simulink model "untitled"  (R2025b)
settings: Solver=VariableStepAuto  StartTime=0.0  StopTime=0.5  FixedStep=1e-5  RelTol=1e-3
libraries: fl_lib x17, nesl_utility x7, eeGeneralControl x2, eePowerMeasurement x1
settings Model: Creator=lenovo  LastModifiedBy=lenovo

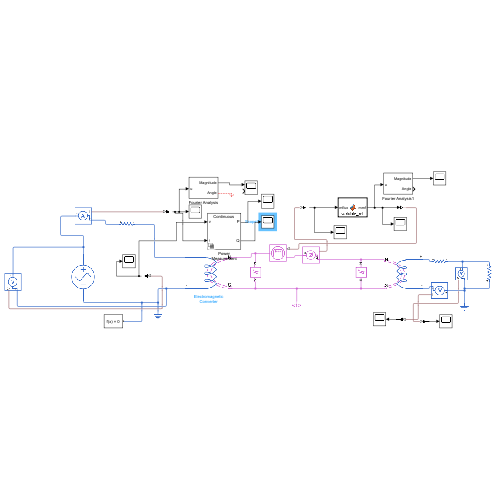
[thumbnail: Simulink's stored preview of the top-level diagram]
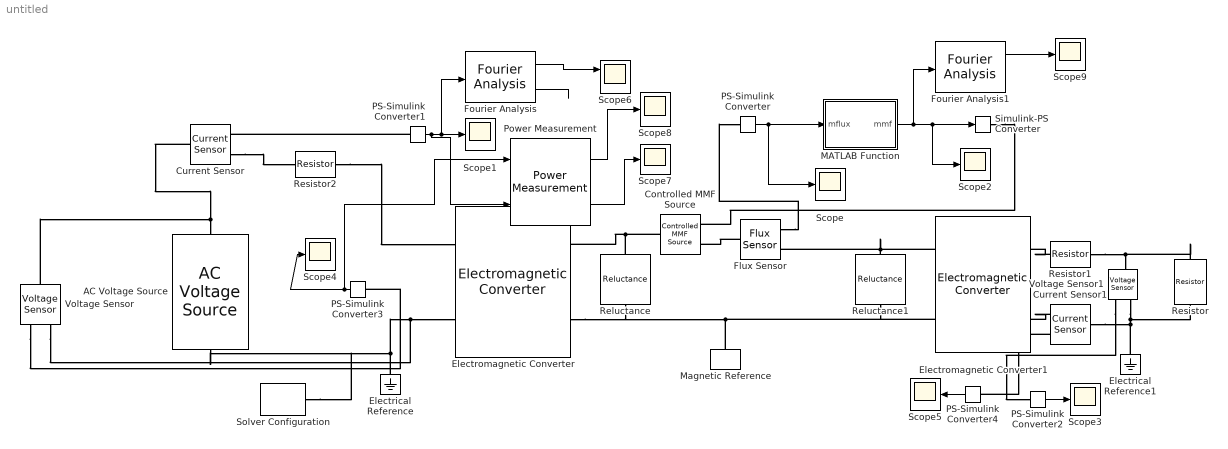
== system untitled ==
  AC Voltage Source : fl_lib/Electrical/Electrical Sources/AC Voltage Source  amp=49.9 V  shift=90 deg  frequency=50 Hz
  Controlled MMF Source : fl_lib/Magnetic/Magnetic Sources/Controlled MMF Source
      settings: InternalSimscapePortConfiguration="{\"Bottom\":[],\"Left\":[{\"id\":\"N\",\"label\":\"\",\"type\":\"foundation.magnetic.magnetic\"}],\"Right\":[{\"id\":\"mmfI\",\"label\":\"\",\"type\":\"input\"},{\"id\":\"S\",\"label\":\"\",\"type\":\"foundation.magnetic.magnetic\"}],\"Top\":[]}"
  Current Sensor : fl_lib/Electrical/Electrical Sensors/Current Sensor
  Current Sensor1 : fl_lib/Electrical/Electrical Sensors/Current Sensor
  Electrical Reference : fl_lib/Electrical/Electrical Elements/Electrical Reference
  Electrical Reference1 : fl_lib/Electrical/Electrical Elements/Electrical Reference
  Electromagnetic Converter : fl_lib/Magnetic/Magnetic Elements/Electromagnetic Converter  Nw=320  i_specify=off  i_priority=None  i=0 A  i_nominal_specify=off  i_nominal_value=1  i_nominal_unit=A  v_specify=off  v_priority=None  v=0 V  v_nominal_specify=off  v_nominal_value=1  v_nominal_unit=V  mmf_specify=off  mmf_priority=None  mmf=0 A  mmf_nominal_specify=off  mmf_nominal_value=1  mmf_nominal_unit=A  phi_specify=off  phi_priority=High  phi=0 Wb  phi_nominal_specify=off  phi_nominal_value=1  phi_nominal_unit=Wb
      settings: InternalSimscapePortConfiguration="{\"Bottom\":[],\"Left\":[{\"id\":\"p\",\"label\":\"+\",\"type\":\"foundation.electrical.electrical\"},{\"id\":\"n\",\"label\":\"-\",\"type\":\"foundation.electrical.electrical\"}],\"Right\":[{\"id\":\"N\",\"label\":\"N\",\"type\":\"foundation.magnetic.magnetic\"},{\"id\":\"S\",\"label\":\"S\",\"type\":\"foundation.magnetic.magnetic\"}],\"Top\":[]}"
  Electromagnetic Converter1 : fl_lib/Magnetic/Magnetic Elements/Electromagnetic Converter  Nw=56  i_specify=off  i_priority=None  i=0 A  i_nominal_specify=off  i_nominal_value=1  i_nominal_unit=A  v_specify=off  v_priority=None  v=0 V  v_nominal_specify=off  v_nominal_value=1  v_nominal_unit=V  mmf_specify=off  mmf_priority=None  mmf=0 A  mmf_nominal_specify=off  mmf_nominal_value=1  mmf_nominal_unit=A  phi_specify=off  phi_priority=High  phi=0 Wb  phi_nominal_specify=off  phi_nominal_value=1  phi_nominal_unit=Wb
      settings: InternalSimscapePortConfiguration="{\"Bottom\":[],\"Left\":[{\"id\":\"p\",\"label\":\"+\",\"type\":\"foundation.electrical.electrical\"},{\"id\":\"n\",\"label\":\"-\",\"type\":\"foundation.electrical.electrical\"}],\"Right\":[{\"id\":\"N\",\"label\":\"N\",\"type\":\"foundation.magnetic.magnetic\"},{\"id\":\"S\",\"label\":\"S\",\"type\":\"foundation.magnetic.magnetic\"}],\"Top\":[]}"
  Flux Sensor : fl_lib/Magnetic/Magnetic Sensors/Flux Sensor
      settings: InternalSimscapePortConfiguration="{\"Bottom\":[],\"Left\":[{\"id\":\"N\",\"label\":\"N\",\"type\":\"foundation.magnetic.magnetic\"}],\"Right\":[{\"id\":\"PHI\",\"label\":\"\",\"type\":\"output\"},{\"id\":\"S\",\"label\":\"S\",\"type\":\"foundation.magnetic.magnetic\"}],\"Top\":[]}"
  Fourier Analysis : eeGeneralControl/Fourier Analysis  f=50  n=[1]  M0=1  Ph0=0  BufferSize=8192  Ts=0
      settings: LibrarySourceBlock=ee_sl_lib/General Control/Fourier Analysis
  Fourier Analysis1 : eeGeneralControl/Fourier Analysis  f=50  n=[1]  M0=1  Ph0=0  BufferSize=8192  Ts=0
      settings: LibrarySourceBlock=ee_sl_lib/General Control/Fourier Analysis
  MATLAB Function : MATLAB Function  TreatAsAtomicUnit=on
  Magnetic Reference : fl_lib/Magnetic/Magnetic Elements/Magnetic Reference
      settings: InternalSimscapePortConfiguration="{\"Bottom\":[],\"Left\":[{\"id\":\"M\",\"label\":\"\",\"type\":\"foundation.magnetic.magnetic\"}],\"Right\":[],\"Top\":[]}"
  PS-Simulink Converter{,1..4} (5 alike) : nesl_utility/PS-Simulink Converter  PhysicalDomain=network_engine_domain  SubClassName=ps_output  LeftPortType=input  RightPortType=output  PseudoPeriodic=off  Frequencies=[]  VectorFormat=inherit  Unit=inherit  AffineConversion=off
  Power Measurement : eePowerMeasurement/Power Measurement  LabelModeActiveChoice=Continuous  F=50  K=[1]  Ts=0
  Reluctance : fl_lib/Magnetic/Magnetic Elements/Reluctance  g=0.1 m  CSA=0.0625 m^2  mur=1  phi_specify=off  phi_priority=None  phi=0 Wb  phi_nominal_specify=off  phi_nominal_value=1  phi_nominal_unit=Wb  mmf_specify=off  mmf_priority=None  mmf=0 A  mmf_nominal_specify=off  mmf_nominal_value=1  mmf_nominal_unit=A
      settings: InternalSimscapePortConfiguration="{\"Bottom\":[],\"Left\":[{\"id\":\"N\",\"label\":\"N\",\"type\":\"foundation.magnetic.magnetic\"}],\"Right\":[{\"id\":\"S\",\"label\":\"S\",\"type\":\"foundation.magnetic.magnetic\"}],\"Top\":[]}"
  Reluctance1 : fl_lib/Magnetic/Magnetic Elements/Reluctance  g=0.1 m  CSA=0.0625 m^2  mur=1  phi_specify=off  phi_priority=None  phi=0 Wb  phi_nominal_specify=off  phi_nominal_value=1  phi_nominal_unit=Wb  mmf_specify=off  mmf_priority=None  mmf=0 A  mmf_nominal_specify=off  mmf_nominal_value=1  mmf_nominal_unit=A
      settings: InternalSimscapePortConfiguration="{\"Bottom\":[],\"Left\":[{\"id\":\"N\",\"label\":\"N\",\"type\":\"foundation.magnetic.magnetic\"}],\"Right\":[{\"id\":\"S\",\"label\":\"S\",\"type\":\"foundation.magnetic.magnetic\"}],\"Top\":[]}"
  Resistor : fl_lib/Electrical/Electrical Elements/Resistor  R=2 mOhm  i_specify=off  i_priority=None  i=0 A  i_nominal_specify=off  i_nominal_value=1  i_nominal_unit=A  v_specify=off  v_priority=None  v=0 V  v_nominal_specify=off  v_nominal_value=1  v_nominal_unit=V
  Resistor1 : fl_lib/Electrical/Electrical Elements/Resistor  R=200 mOhm  i_specify=off  i_priority=None  i=0 A  i_nominal_specify=off  i_nominal_value=1  i_nominal_unit=A  v_specify=off  v_priority=None  v=0 V  v_nominal_specify=off  v_nominal_value=1  v_nominal_unit=V
  Resistor2 : fl_lib/Electrical/Electrical Elements/Resistor  R=8 Ohm  i_specify=off  i_priority=None  i=0 A  i_nominal_specify=off  i_nominal_value=1  i_nominal_unit=A  v_specify=off  v_priority=None  v=0 V  v_nominal_specify=off  v_nominal_value=1  v_nominal_unit=V
  Scope{,1..5,7..9} (9 alike) : Scope
      Scope settings: ActiveDisplayYMinimum=-0.0040423154609422968  ActiveDisplayYMaximum=0.0040377042195075428
      Scope1 settings: ActiveDisplayYMinimum=-1.2684889472034619  ActiveDisplayYMaximum=1.1956642559367752
      Scope2 settings: ActiveDisplayYMinimum=-26.473084581428164  ActiveDisplayYMaximum=26.303381950639405  DataLoggingVariableName=ScopeData2
      Scope3 settings: ActiveDisplayYMinimum=-1  ActiveDisplayYMaximum=1  DataLoggingVariableName=ScopeData3
      Scope4 settings: ActiveDisplayYMinimum=-406.20609199284195  ActiveDisplayYMaximum=406.5440102214269  DataLoggingVariableName=ScopeData4
      Scope5 settings: ActiveDisplayYMinimum=-1  ActiveDisplayYMaximum=1  DataLoggingVariableName=ScopeData5
      Scope7 settings: ActiveDisplayYMinimum=0.44389028789857221  ActiveDisplayYMaximum=23.400654164800176  DataLoggingVariableName=ScopeData7
      Scope8 settings: ActiveDisplayYMinimum=0.19457580868154878  ActiveDisplayYMaximum=9.3781897944855732  DataLoggingVariableName=ScopeData8
      Scope9 settings: ActiveDisplayYMinimum=-26.473084581428164  ActiveDisplayYMaximum=26.303381950639405  DataLoggingVariableName=ScopeData9
  Scope6 : Scope  NumInputPorts=2
      settings: ActiveDisplayYMinimum=-0.12499999999999997  ActiveDisplayYMaximum=1.125  DataLoggingVariableName=ScopeData6
  Simulink-PS Converter : nesl_utility/Simulink-PS Converter  PhysicalDomain=network_engine_domain  SubClassName=ps_input  LeftPortType=input  RightPortType=output  PseudoPeriodic=off  Frequencies=[]  NoiseDistribution=none  NoiseParameters=[]  Unit=1  AffineConversion=off  FilteringAndDerivatives=provide  SimscapeFilterOrder=1  InputFilterTimeConstant=0.001  UdotUserProvided=0
  Solver Configuration : nesl_utility/Solver Configuration  PhysicalDomain=network_engine_domain  SubClassName=solver  LeftPortType=input  RightPortType=generic  Tones=[]  Harmonics=[]  SimulateNoise=off  Profile=off  UseLocalSampling=off  EnableSwitchedLinearOptims=on  FrequencyDomain=off  UseCCode=off  RelTol=0.001  AbsTol=0.001  MinStep=1e-09  ToWorkspace=off  RevertToSquareIcSolve=off  NumHomotopyIterations=100  PhasorMode=off  PhasorModeNumHarmonics=1  ConsistencySolver=NEWTON_XTOL_AFTER_FTOL  IndexReductionMethod=DerivativeReplacement  DoDC=off  ResidualTolerance=1e-09  ConsistencyTolSource=GLOBAL  ConsistencyAbsTol=0.001  ConsistencyRelTol=0.001  ConsistencyTolFactor=0.001  UseLocalSolver=off  LocalSolverChoice=NE_BACKWARD_EULER_ADVANCER  ResolveIndetEquations=on  FunctionEvalNumThread=1  LocalSolverSampleTime=0.001  DoFixedCost=off  MaxNonlinIter=3  MaxModeIter=2  ComputeImpulses=off  ImpulseIterations=2  LinearAlgebra=auto  LinearAlgebraNumThread=0  EquationFormulation=NE_TIME_EF  DelaysMemoryBudget=1024  AutomaticFiltering=on  FilteringTimeConstant=0.001  PartitionStorageMethod=AS_NEEDED  PartitionMemoryBudget=1024  PartitionMethod=ROBUST  MultibodyUseLocalSolver=off  MultibodyLocalSolverChoice=ODE1  MultibodyLocalSolverSampleTime=0.001
  Voltage Sensor : fl_lib/Electrical/Electrical Sensors/Voltage Sensor
  Voltage Sensor1 : fl_lib/Electrical/Electrical Sensors/Voltage Sensor
  wires:
  MATLAB Function/1(mmf) -> Fourier Analysis1/1, Scope2/1, Simulink-PS Converter/1
  PS-Simulink Converter1/1 -> Power Measurement/2, Fourier Analysis/1, Scope1/1
  PS-Simulink Converter/1 -> Scope/1, MATLAB Function/1(mflux)
  PS-Simulink Converter2/1 -> Scope3/1
  PS-Simulink Converter3/1 -> Power Measurement/1, Scope4/1
  PS-Simulink Converter4/1 -> Scope5/1
  Fourier Analysis/1 -> Scope6/1
  Power Measurement/2 -> Scope7/1
  Fourier Analysis/2 -> ?
  Power Measurement/1 -> Scope8/1
  Fourier Analysis1/1 -> Scope9/1
  connections:
  Electrical Reference1/LConn1 -- Voltage Sensor1/RConn2 -- Resistor/LConn1 -- Current Sensor1/LConn1
  Electrical Reference/LConn1 -- AC Voltage Source/RConn1 -- Solver Configuration/RConn1 -- Electromagnetic Converter/LConn2 -- Voltage Sensor/RConn2
  Magnetic Reference/LConn1 -- Reluctance/RConn1 -- Electromagnetic Converter/RConn2 -- Reluctance1/RConn1 -- Electromagnetic Converter1/RConn2
  Simulink-PS Converter/RConn1 -- Controlled MMF Source/RConn1
  PS-Simulink Converter1/LConn1 -- Current Sensor/RConn1
  Electromagnetic Converter1/RConn1 -- Reluctance1/LConn1 -- Flux Sensor/RConn2
  Flux Sensor/RConn1 -- PS-Simulink Converter/LConn1
  Resistor/RConn1 -- Resistor1/RConn1 -- Voltage Sensor1/LConn1
  Voltage Sensor1/RConn1 -- PS-Simulink Converter2/LConn1
  Voltage Sensor/RConn1 -- PS-Simulink Converter3/LConn1
  Flux Sensor/LConn1 -- Controlled MMF Source/RConn2
  Controlled MMF Source/LConn1 -- Reluctance/LConn1 -- Electromagnetic Converter/RConn1
  Resistor1/LConn1 -- Electromagnetic Converter1/LConn1
  AC Voltage Source/LConn1 -- Current Sensor/LConn1 -- Voltage Sensor/LConn1
  Current Sensor1/RConn2 -- Electromagnetic Converter1/LConn2
  Current Sensor1/RConn1 -- PS-Simulink Converter4/LConn1
  Current Sensor/RConn2 -- Resistor2/LConn1
  Resistor2/RConn1 -- Electromagnetic Converter/LConn1

== matlab function untitled/MATLAB Function ==
  data: mflux input; mmf output
function mmf = variable_rel(mflux)
    % Parameters
    A = 36 * 10^(-4);    % Area in m^2
    Length = 0.54;       % Length in meters
    
    % 1. Calculate Flux Density (B = Phi / A)
    B = abs(mflux) / A; 
    
    H = 0.1431 * exp(6.253 * B) - 0.1431;
    mmf = H * Length * sign(mflux);
end
